simulink model "tcs_CS2017"  (Simulink 7.4)
settings: Solver=ode45  SolverMode=SingleTasking  StartTime=0  StopTime=28  FixedStep=0.002  RelTol=1e-3  AbsTol=1e-6
libraries: Solver_SF x1
settings Model: Creator=ywata  LastModifiedBy=ywata  ExtModeTrigMode=oneshot  ExtModeArmWhenConnect=off
settings DataIOCC: LimitDataPoints=off  SignalLoggingName=sigsOut
settings OptimizationCC: BlockReduction=off  BooleanDataType=off
settings DebuggingCC: SaveWithParameterizedLinksMsg=none  SignalResolutionControl=TryResolveAllWithWarning  SolverPrmCheckMsg=none  MultiTaskDSMMsg=warning  MultiTaskCondExecSysMsg=none  StrictBusMsg=None
settings HardwareCC: TargetUnknown=on
settings RTWCC: TemplateMakefile=grt_vc.tmf  IncludeERTFirstTime=on
settings GRTTargetCC: TargetFcnLib=ansi_tfl_tmw.mat

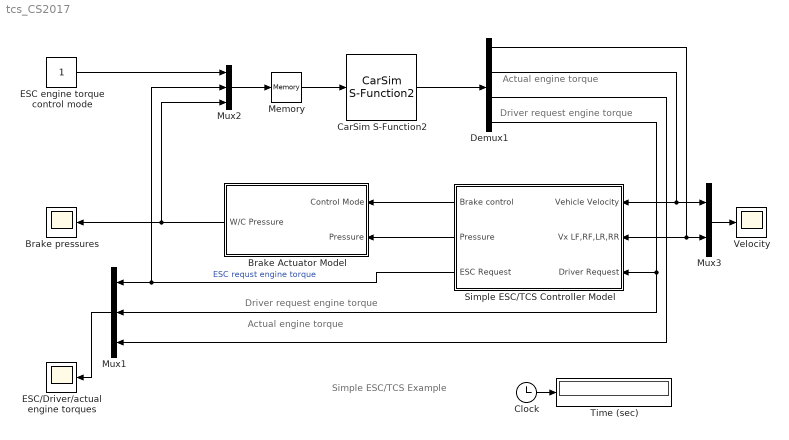
== system tcs_CS2017 ==
  note: Simple ESC/TCS Example
  note: Actual engine torque
  note: Actual engine torque
  note: Driver request engine torque
  note: Driver request engine torque
  Brake Actuator Model : Subsystem
  Brake pressures : Scope
      settings: TickLabels=on  YMin=0  YMax=8  SaveName=ScopeData2  DataFormat=Array  SampleTime=100
  CarSim S-Function2 : Solver_SF/CarSim S-Function2  Priority=1  VehicleCode=i_i  SIMFILE=simfile.sim
      settings: AttributesFormatString=Vehicle Code: %<VehicleCode>
  Clock : Clock
      settings: Decimation=10
  Demux1 : Demux  Outputs=[4 1 1 1]
  ESC engine torque control mode : Constant  OutDataType=fixdt(1, 16)  OutScaling=2^0
  ESC/Driver/actual engine torques : Scope
      settings: TickLabels=on  YMin=0  YMax=800  DataFormat=Array  SampleTime=100
  Memory : Memory
  Mux1 : Mux  Inputs=3
  Mux2 : Mux  Inputs=3
  Mux3 : Mux  Inputs=2
  Simple ESC/TCS Controller Model : Subsystem
  Time (sec) : Display
      settings: Format=bank  Decimation=100
  Velocity : Scope
      settings: TickLabels=on  TimeRange=28  YMin=-10  YMax=250  DataFormat=Array  SampleTime=100
  wires:
  CarSim S-Function2/1 -> Demux1/1
  Demux1/2 -> Mux3/1, Simple ESC/TCS Controller Model/1(Vehicle Velocity)
  Clock/1 -> Time (sec)/1
  Mux3/1 -> Velocity/1
  Simple ESC/TCS Controller Model/1(Brake control) -> Brake Actuator Model/1(Control Mode)
  Memory/1 -> CarSim S-Function2/1
  Mux1/1 -> ESC/Driver/actual engine torques/1
  Mux2/1 -> Memory/1
  ESC engine torque control mode/1 -> Mux2/1
  Demux1/4 -> Mux1/2, Simple ESC/TCS Controller Model/3(Driver Request)
  Demux1/3 -> Mux1/3
  Simple ESC/TCS Controller Model/2(Pressure) -> Brake Actuator Model/2(Pressure)
  Brake Actuator Model/1(W/C Pressure) -> Mux2/3, Brake pressures/1
  Simple ESC/TCS Controller Model/3(ESC Request) -> Mux2/2, Mux1/1  "ESC requst engine torque"
  Demux1/1 -> Simple ESC/TCS Controller Model/2(Vx LF,RF,LR,RR), Mux3/2

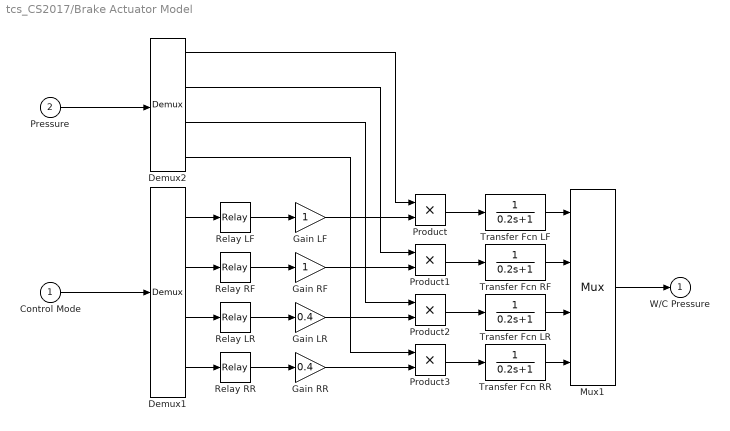
== system tcs_CS2017/Brake Actuator Model ==
  Control Mode : Inport
  Pressure : Inport  Port=2
  Demux1 : Demux
  Demux2 : Demux
  Gain LF : Gain  SaturateOnIntegerOverflow=on  OutDataTypeStr=Inherit: Same as input  ParamDataTypeStr=Inherit: Same as input
  Gain LR : Gain  Gain=0.4  SaturateOnIntegerOverflow=on  OutDataTypeStr=Inherit: Same as input  ParamDataTypeStr=Inherit: Same as input
  Gain RF : Gain  SaturateOnIntegerOverflow=on  OutDataTypeStr=Inherit: Same as input  ParamDataTypeStr=Inherit: Same as input
  Gain RR : Gain  Gain=0.4  SaturateOnIntegerOverflow=on  OutDataTypeStr=Inherit: Same as input  ParamDataTypeStr=Inherit: Same as input
  Mux1 : Mux
  Product{,1..3} (4 alike) : Product  SaturateOnIntegerOverflow=on  RndMeth=Zero  InputSameDT=on  OutDataTypeStr=Inherit: Same as first input
  Relay LF : Relay  OnSwitchValue=0.5  OffSwitchValue=-0.5
  Relay LR : Relay  OnSwitchValue=0.5  OffSwitchValue=-0.5
  Relay RF : Relay  OnSwitchValue=0.5  OffSwitchValue=-0.5
  Relay RR : Relay  OnSwitchValue=0.5  OffSwitchValue=-0.5
  Transfer Fcn LF : TransferFcn  Denominator=[0.2 1]
  Transfer Fcn LR : TransferFcn  Denominator=[0.2 1]
  Transfer Fcn RF : TransferFcn  Denominator=[0.2 1]
  Transfer Fcn RR : TransferFcn  Denominator=[0.2 1]
  W/C Pressure : Outport  InitialOutput=0
  wires:
  Mux1/1 -> W/C Pressure/1
  Control Mode/1 -> Demux1/1
  Demux1/1 -> Relay LF/1
  Demux1/2 -> Relay RF/1
  Demux1/3 -> Relay LR/1
  Demux1/4 -> Relay RR/1
  Relay LF/1 -> Gain LF/1
  Relay RF/1 -> Gain RF/1
  Relay LR/1 -> Gain LR/1
  Relay RR/1 -> Gain RR/1
  Gain LF/1 -> Product/2
  Gain RF/1 -> Product1/2
  Gain LR/1 -> Product2/2
  Gain RR/1 -> Product3/2
  Product/1 -> Transfer Fcn LF/1
  Transfer Fcn LF/1 -> Mux1/1
  Product1/1 -> Transfer Fcn RF/1
  Product2/1 -> Transfer Fcn LR/1
  Product3/1 -> Transfer Fcn RR/1
  Transfer Fcn RF/1 -> Mux1/2
  Transfer Fcn LR/1 -> Mux1/3
  Transfer Fcn RR/1 -> Mux1/4
  Pressure/1 -> Demux2/1
  Demux2/4 -> Product3/1
  Demux2/3 -> Product2/1
  Demux2/2 -> Product1/1
  Demux2/1 -> Product/1

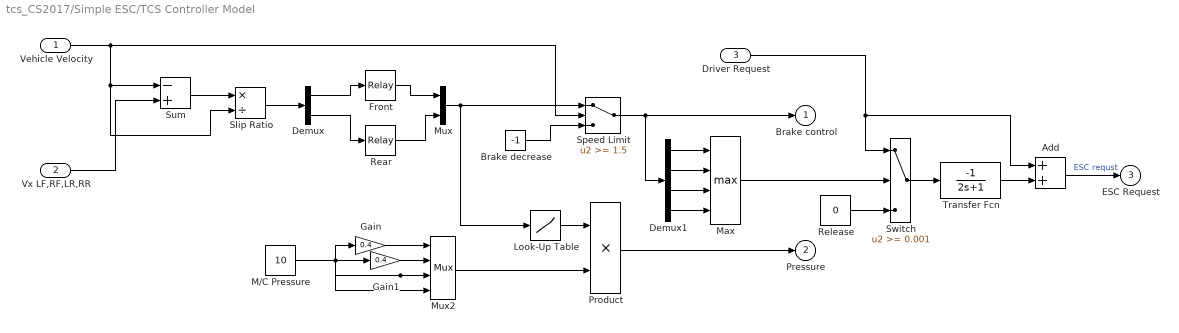
== system tcs_CS2017/Simple ESC/TCS Controller Model ==
  Vehicle Velocity : Inport  OutDataType=sfix(16)  OutScaling=2^0
  Vx LF,RF,LR,RR : Inport  Port=2  OutDataType=sfix(16)  OutScaling=2^0
  Driver Request : Inport  Port=3  OutDataType=sfix(16)  OutScaling=2^0
  Add : Sum  OutDataType=fixdt(1, 16)  OutScaling=2^-10
  Brake decrease : Constant  Value=-1  OutDataType=sfix(16)  OutScaling=2^0
  Demux : Demux  Outputs=[2 2]
  Demux1 : Demux
  Front : Relay  OnSwitchValue=0.1  OffSwitchValue=0.05  OffOutputValue=-1  OutDataType=sfix(16)  OutScaling=2^0
  Gain : Gain  Gain=0.4  SaturateOnIntegerOverflow=on  OutDataTypeStr=Inherit: Same as input  ParamDataTypeStr=Inherit: Same as input
  Gain1 : Gain  Gain=0.4  SaturateOnIntegerOverflow=on  OutDataTypeStr=Inherit: Same as input  ParamDataTypeStr=Inherit: Same as input
  Look-Up Table : Lookup  InputValues=[-1,0,0.01,0.05,1,2]  Table=[0,0,0.2,0.2,1.5,1.5]  SaturateOnIntegerOverflow=on
  M/C Pressure : Constant  Value=10
  Max : MinMax  Function=max  Inputs=4  SaturateOnIntegerOverflow=on  InputSameDT=on
  Mux : Mux  Inputs=2
  Mux2 : Mux
  Product : Product  SaturateOnIntegerOverflow=on  RndMeth=Zero  InputSameDT=on  OutDataTypeStr=Inherit: Same as first input
  Rear : Relay  OnSwitchValue=0.1  OffSwitchValue=0.05  OffOutputValue=-1  OutDataType=sfix(16)  OutScaling=2^0
  Release : Constant  Value=0  OutDataType=fixdt(1, 16)  OutScaling=2^0
  Slip Ratio : Product  Inputs=*/  OutDataType=sfix(16)  OutScaling=2^0  SaturateOnIntegerOverflow=on  InputSameDT=on  OutDataTypeStr=Inherit: Same as first input
  Speed Limit : Switch  Threshold=1.5  SaturateOnIntegerOverflow=on  InputSameDT=on
  Sum : Sum  Inputs=-+  OutDataType=sfix(16)  OutScaling=2^0  SaturateOnIntegerOverflow=on  InputSameDT=on  OutDataTypeStr=Inherit: Same as first input
  Switch : Switch  Threshold=0.001  OutDataType=fixdt(1, 16)  OutScaling=2^0
  Transfer Fcn : TransferFcn  Numerator=[-1]  Denominator="[2  1]"
  Brake control : Outport  InitialOutput=0
  Pressure : Outport  Port=2  InitialOutput=0
  ESC Request : Outport  Port=3  InitialOutput=0
  wires:
  Vehicle Velocity/1 -> Sum/1, Slip Ratio/2, Speed Limit/2
  Brake decrease/1 -> Speed Limit/3
  Sum/1 -> Slip Ratio/1
  Slip Ratio/1 -> Demux/1
  Mux/1 -> Speed Limit/1, Look-Up Table/1
  Demux1/2 -> Max/2
  Demux1/1 -> Max/1
  Front/1 -> Mux/1
  Demux/1 -> Front/1
  Demux/2 -> Rear/1
  Rear/1 -> Mux/2
  Vx LF,RF,LR,RR/1 -> Sum/2
  Demux1/3 -> Max/3
  Demux1/4 -> Max/4
  Look-Up Table/1 -> Product/1
  Product/1 -> Pressure/1
  Mux2/1 -> Product/2
  M/C Pressure/1 -> Mux2/3, Mux2/4, Gain1/1, Gain/1
  Gain1/1 -> Mux2/2
  Gain/1 -> Mux2/1
  Speed Limit/1 -> Brake control/1, Demux1/1
  Switch/1 -> Transfer Fcn/1
  Max/1 -> Switch/2
  Driver Request/1 -> Switch/1, Add/1
  Release/1 -> Switch/3
  Transfer Fcn/1 -> Add/2
  Add/1 -> ESC Request/1  "ESC requst"
